simulink model "ekf_estimation_mass_slope"  (R2021a)
settings: Solver=VariableStepAuto  StartTime=0.0  StopTime=10.0  RelTol=1e-3
settings Model: Creator=huawei  LastModifiedBy=huawei

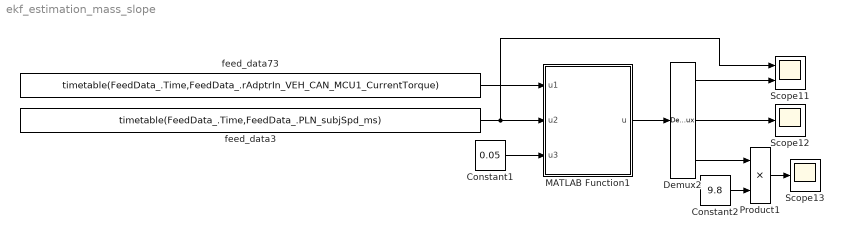
== system ekf_estimation_mass_slope ==
  Constant1 : Constant  Value=0.05
  Constant2 : Constant  Value=9.8
  Demux2 : Demux  Outputs=3
      settings: DisplayOption=none
  MATLAB Function1 : MATLAB Function  TreatAsAtomicUnit=on
  Product1 : Product
  Scope11 : Scope  NumInputPorts=2
  Scope12 : Scope
  Scope13 : Scope
  feed_data3 : FromWorkspace  VariableName=timetable(FeedData_.Time,FeedData_.PLN_subjSpd_ms)  Interpolate=off  OutputAfterFinalValue=Holding final value
  feed_data73 : FromWorkspace  VariableName=timetable(FeedData_.Time,FeedData_.rAdptrIn_VEH_CAN_MCU1_CurrentTorque)  Interpolate=off  OutputAfterFinalValue=Holding final value
  wires:
  Constant2/1 -> Product1/2
  Product1/1 -> Scope13/1
  Demux2/3 -> Product1/1
  Demux2/2 -> Scope12/1
  feed_data73/1 -> MATLAB Function1/1(u1)
  feed_data3/1 -> Scope11/1, MATLAB Function1/2(u2)
  MATLAB Function1/1(u) -> Demux2/1
  Demux2/1 -> Scope11/2
  Constant1/1 -> MATLAB Function1/3(u3)

== matlab function ekf_estimation_mass_slope/MATLAB Function1 ==
  data: u1 input; u output; u2 input; u3 input

function u = EKF_estimatd(u1,u2,u3)
%u1:输入Ttq
Ttq=u1;
%u2:系统噪声W
z=u2;
%u3:时间t
t=u3;

%persistent v m i
persistent x  P V0

    Ts=0.1;
    ig=1.0;
    i0=6.83;
    nn=0.95*0.96;
    g=9.8;
    f=0.011;
    r=0.502;
    CD=0.65;%%%%%卡车取0.8 客车0.65
    A=1.92*3.09;
    rou=1.2258;
    qq=1.027+0.000331*i0^2.*ig.^2;%%汽车质量转换系数
    
    %系统方程：
    
    H=[1.0,0.0,0.0];  
      
    %Covariances of w:
    Q=diag([Ts*0.1*Ts',0.0,0.001]);

    %Covariances of v:
    R=[0.1];

    %初始估计值：
    if isempty(x)
        x=[0;3000;0.0];
        %初始估计误差协方差：
        P=diag([Ts*0.1*Ts',9000000000,0.000001]);
    end
    if isempty(V0)
       V0 = 0; 
    end
    
    u=x;%开始时刻不进行卡尔曼滤波，直接将初始值输出,2020


   %%卡尔曼滤波：：

    %先验，Time update:
    %根据系统状态方程计算下一状态预测值：
    %x=A*x+B*u1;
    Jf=eye(3);
    Jf(1,1)=1-CD*A*rou*x(1)*Ts/x(2)/qq;%add /qq 2020
    Jf(1,2)=(CD*A*rou*x(1)^2*r-2*Ttq*ig*i0*nn)/(2*x(2)^2*r)*Ts/qq;%add /qq 2020
    Jf(1,3)=-g*Ts; 

    v=x(1);
    m=x(2);
    i=x(3);
    dv=1/qq*(Ttq*ig*i0*nn/(m*r)-g*f-CD*A*rou*v^2/(2*m)-g*i);
    v=v+Ts*dv;
    x(1)=v;
    x(2)=m;
    x(3)=i;
 
    %************强跟踪滤波器STF核心代码《：：*********************************
    %**************************************
    % 可调节参数汇总
    %**************************************
    rho=0.95;                         % 残差方差阵的遗忘因子初始值 (0.95<rho<0.995)
    beta=1;                           % 量测噪声的衰减因子选定值 (beta>=1)
    %beta_upmax=8;                     % 衰减因子选定极限
    %***************************************
    F=Jf;
    r0=z-H*x;
    if t==Ts
        V0=r0*r0';
    else
        V0=(rho*V0+r0*r0')/(1+rho);
    end
    N=V0-beta*R-H*Q*H';
    M=H*F*P*F'*H';
    eta=trace(N)/trace(M);
    if eta>1
        lamda=eta;
    else
        lamda=1;
    end
    
    %预测误差协方差：
    P=lamda*Jf*P*Jf'+Q;  
    %！！！渐消因子lamda=1即为普通卡尔曼滤波！！！
    %************STF核心代码》************************************************
    
    %后验，Measurement update:
    %根据估计误差协方差和测量噪声协方差计算卡尔曼增益：
    Kk=P*H'/(H*P*H'+R);

    %计算最优估计值：    
    %x=A*x+Mn*(yv-C*A*x);
    x=x+Kk*(z-H*x);

    %计算最优估计值和真实值之间的误差协方差矩阵，为下次递推做准备：
    P=(eye(3)-Kk*H)*P;

    %ye=C*x;           %Filtered value
    u=x;    %Filtered signal

    errcov=H*P*H';      %Covariance of estimation error   
    
end
%}
